simulink model "SimpleReverb"  (R2023b)
settings: Solver=VariableStepAuto  StartTime=0.0  StopTime=inf  RelTol=1e-3
libraries: dspsrcs4 x1
settings Model: Creator=shaanyadav  LastModifiedBy=shaanyadav

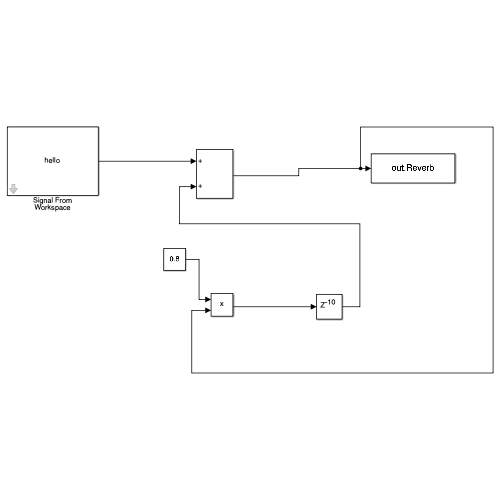
[thumbnail: Simulink's stored preview of the top-level diagram]
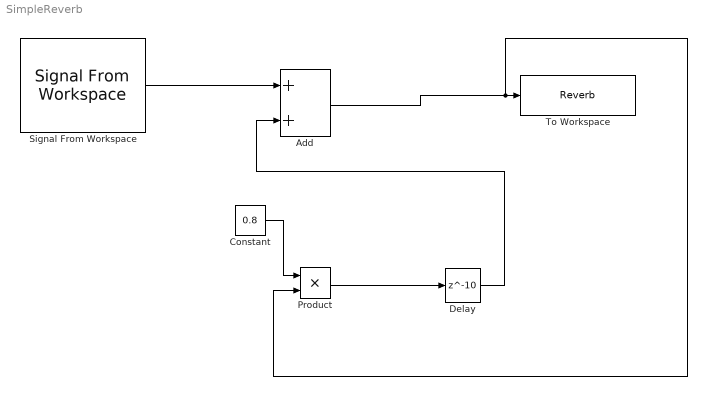
== system SimpleReverb ==
  Add : Sum
  Constant : Constant  Value=0.8
  Delay : Delay  DelayLength=10  InitialCondition=0
  Product : Product
  Signal From Workspace : dspsrcs4/Signal From Workspace  X=hello  Ts=1/8000  nsamps=64  OutputAfterFinalValue=Setting to zero  ignoreOrWarnInputAndFrameLengths=off  OutputFrames=off
  To Workspace : ToWorkspace  VariableName=Reverb  SampleTime=-1
      settings: Save2DSignal=2-D array (concatenate along first dimension)
  wires:
  Add/1 -> Product/2, To Workspace/1
  Delay/1 -> Add/2
  Signal From Workspace/1 -> Add/1
  Constant/1 -> Product/1
  Product/1 -> Delay/1
